simulink model "GFLIB_Lut1D_BAM"  (Simulink 9.3)
settings: Solver=VariableStepAuto  StartTime=0.0  StopTime=10.0  RelTol=1e-3
settings Model: Creator=nxa18952  LastModifiedBy=nxa18952
settings DataIOCC: SaveFormat=Dataset  SignalLoggingSaveFormat=Dataset  ReturnWorkspaceOutputs=on
settings OptimizationCC: LifeSpan=auto
settings DebuggingCC: UnderspecifiedInitializationDetection=Simplified  MergeDetectMultiDrivingBlocksExec=error  FcnCallInpInsideContextMsg=error  SFUnexpectedBacktrackingDiag=error  SFNoUnconditionalDefaultTransitionDiag=error  SFExecutionAtInitializationDiag=warning  ArithmeticOperatorsInVariantConditions=error
settings HardwareCC: ProdBitPerPointer=64  ProdBitPerSizeT=64  ProdBitPerPtrDiffT=64  ProdLargestAtomicFloat=Float  ProdIntDivRoundTo=Zero  ProdEndianess=LittleEndian  ProdWordSize=64  ProdHWDeviceType=Intel->x86-64 (Windows64)
settings ModelReferenceCC: PropagateSignalLabelsOutOfModel=on
settings SFSimCC: SimUseLocalCustomCode=on
settings RTWCC: RTWUseLocalCustomCode=on
settings CodeAppCC: StateflowObjectComments=off
settings GRTTargetCC: TargetLangStandard=C99 (ISO)  CombineOutputUpdateFcns=on  GRTInterface=off
settings ConfigComp: CovMetricSettings=dwe  CovHtmlReporting=off  CovSaveCumulativeToWorkspaceVar=off  CovSaveSingleToWorkspaceVar=off  CovExternalEMLEnable=on

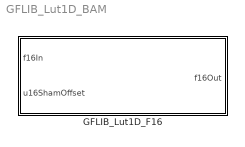
== system GFLIB_Lut1D_BAM ==
  GFLIB_Lut1D_F16 : Subsystem  TreatAsAtomicUnit=on  mask(GFLIB_Lut1D_F16){pf16Table=2^15*[-0.75 -0.25 0.0 0.25 0.75], s16MidIdx=2}
      mask prompts: pf16Table "pf16Table (Vector holding the ordinate values of interpolating intervals)"; s16MidIdx "Middle index in the table pf16Table (zero-based indexing)"
      mask help: One dimensional lookup table function in 16-bit fixed-point fractional implementation. Refer to the AMMCLIB User's Guide for further details.
      mask init:
      | if ~evalin('base','exist(''tS8'',''var'')')
      |   if (2 ~= exist('SWLIBS_Typedefs.mat','file'))
      |       error('File SWLIBS_Typedefs.mat is not on the Matlab path. Please add the AMMCLIB "bam" folder in the Matlab Search Path.');
      |   else
      |       evalin('base', 'load(''SWLIBS_Typedefs.mat'')');
      |   end
      | end
      settings: RTWSystemCode=Inline
      mask Display: pos = get_param(gcb, 'Position');width = pos(3) - pos(1); height = pos(4) - pos(2);tX=width/2;tY=height - 8;color('black');text(tX,tY, 'GFLIB_Lut1D_F16', 'horizontalAlignment', 'center');

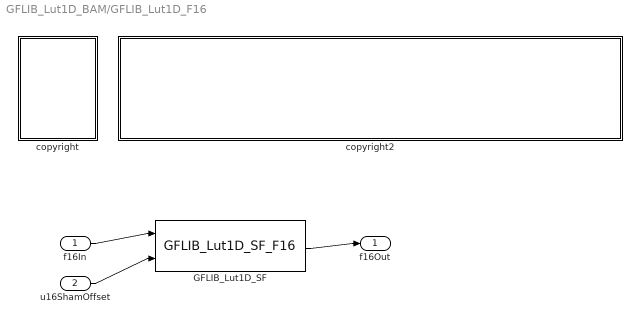
== system GFLIB_Lut1D_BAM/GFLIB_Lut1D_F16 ==
  f16In : Inport  OutDataTypeStr=int16
  u16ShamOffset : Inport  Port=2  OutDataTypeStr=uint16
  GFLIB_Lut1D_SF : S-Function  FunctionName=GFLIB_Lut1D_SF_F16  Parameters=pf16Table,s16MidIdx  SFunctionDeploymentMode=off  EnableBusSupport=off
  copyright : Subsystem
      mask Display: text(10,90,'FILE:');text(10,75,'DESRIPTION:');text(10,60,'COPYRIGHT:');text(10,45,'VERSION:');text(10,30,'DATE:')
  copyright2 : Subsystem
      mask Display: text(10,90,'GFLIB_Lut1D_BAM_F16.mdl');text(10,75,'One dimensional lookup table function');text(10,60,'NXP 2020');text(10,45,'1.0');text(10,30,'23-Mar-2020');
  f16Out : Outport
  wires:
  f16In/1 -> GFLIB_Lut1D_SF/1
  u16ShamOffset/1 -> GFLIB_Lut1D_SF/2
  GFLIB_Lut1D_SF/1 -> f16Out/1

== system GFLIB_Lut1D_BAM/GFLIB_Lut1D_F16/copyright ==

== system GFLIB_Lut1D_BAM/GFLIB_Lut1D_F16/copyright2 ==
